simulink model "Q2_sim2"  (R2023b)
settings: Solver=VariableStepAuto  StartTime=0.0  StopTime=7  RelTol=1e-3
settings Model: Creator=avikd  LastModifiedBy=avikd

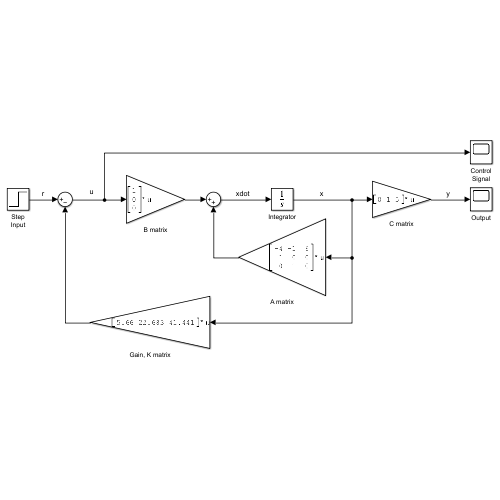
[thumbnail: Simulink's stored preview of the top-level diagram]
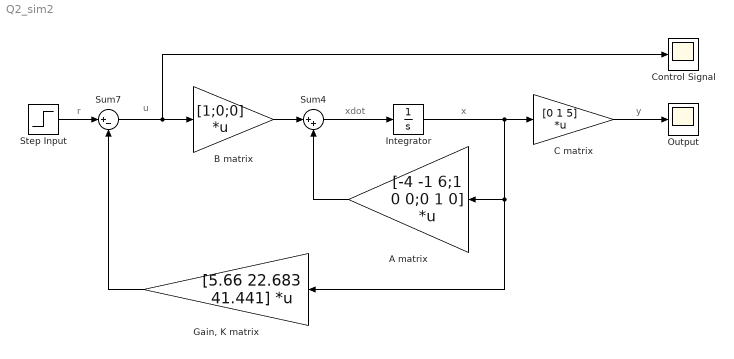
== system Q2_sim2 ==
  note: x
  note: xdot
  note: u
  note: y
  note: r
  A matrix : Gain  Gain=[-4 -1 6;1 0 0;0 1 0]  Multiplication=Matrix(K*u)
  B matrix : Gain  Gain=[1;0;0]  Multiplication=Matrix(K*u)
  C matrix : Gain  Gain=[0 1 5]  Multiplication=Matrix(K*u)
  Control Signal : Scope
  "Gain, K matrix" : Gain  Gain=[5.66 22.683 41.441]  Multiplication=Matrix(K*u)
  Integrator : Integrator
  Output : Scope
  Step Input : Step  Time=0  SampleTime=0
  Sum4 : Sum  Inputs=|++
  Sum7 : Sum  Inputs=|+-
  wires:
  Sum7/1 -> Control Signal/1, B matrix/1
  C matrix/1 -> Output/1
  A matrix/1 -> Sum4/2
  "Gain, K matrix"/1 -> Sum7/2
  Integrator/1 -> C matrix/1, "Gain, K matrix"/1, A matrix/1
  B matrix/1 -> Sum4/1
  Step Input/1 -> Sum7/1
  Sum4/1 -> Integrator/1
